simulink model "ece456hw61c"  (R2017a)
settings: Solver=VariableStepAuto  StartTime=0.0  StopTime=10.0  RelTol=1e-3
values from neighbouring files (symbols this model uses):
  kb = .4953    (= 0.4953)    [ece456hw5.m]    (also in ece456hw6.m)
  ke = .3234    (= 0.3234)    [ece456hw5.m]    (also in ece456hw6.m)
  R = 1000    [ece456hw5.m]    (also in ece456hw6.m = 4.67; ece456hw8.m = 0.0721)
  T = 4    [ece456hw5.m]    (also in ece456hw6.m = 0.001; ece456hw8.m = 1.98196948682)
libraries: dspsrcs4 x1
settings Model: Creator=b  LastModifiedBy=b

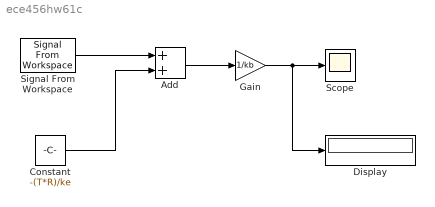
== system ece456hw61c ==
  Add : Sum
  Constant : Constant  Value=-(T*R)/ke
  Display : Display
  Gain : Gain  Gain=1/kb
  Scope : Scope
  Signal From Workspace : dspsrcs4/Signal From Workspace  X=V  Ts=1  nsamps=1  OutputAfterFinalValue=Setting to zero  ignoreOrWarnInputAndFrameLengths=off  OutputFrames=off
  wires:
  Signal From Workspace/1 -> Add/1
  Constant/1 -> Add/2
  Add/1 -> Gain/1
  Gain/1 -> Display/1, Scope/1
